simulink model "balancingOptTauQpExtWrenches"  (Simulink 8.3)
settings: Solver=FixedStepDiscrete  StartTime=0.0  StopTime=simulationTime  FixedStep=Ts  RelTol=1e-3
InitFcn:
  | initBalancingOptTauQpExtWrenches;
values from neighbouring files (symbols this model uses):
  activeFeetConstraints = [1 1]    [initBalancingOptTauQpExtWrenches.m]
  noOscillationTime = 0    [initBalancingOptTauQpExtWrenches.m]
  Ts = 0.01    [initBalancingOptTauQpExtWrenches.m]
undefined symbols (not defined in the file or in its folder): bVectorConstraints, ConstraintsMatrix, dampings, directionOfOscillation, DiscIntNeverNeededParam, footSize, gainMomentum, gainsDCOM, gainsICOM, gainsPCOM, impedances, impedencesSat, increasingRatesImp, integralGains, referenceParams, ROBOT_DOF, ROBOT_DOF_FOR_SIMULINK, satIntegral
undefined symbols (not defined in the file): localName, robotName
libraries: WBCLibrary x35, simulink x2
settings Model: Creator=daniele  LastModifiedBy=daniele
settings DataIOCC: SignalLoggingSaveFormat=Dataset
settings OptimizationCC: ExpressionDepthLimit=2147483647
settings DebuggingCC: FcnCallInpInsideContextMsg=EnableAllAsWarning
settings SFSimCC: SimParseCustomCode=off

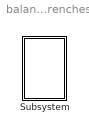
== system balancingOptTauQpExtWrenches ==
  Subsystem : Subsystem  mask{robotName=robotName, Ts=Ts, localName=localName}
      mask prompts: robotName "robot name"; localName "module name"

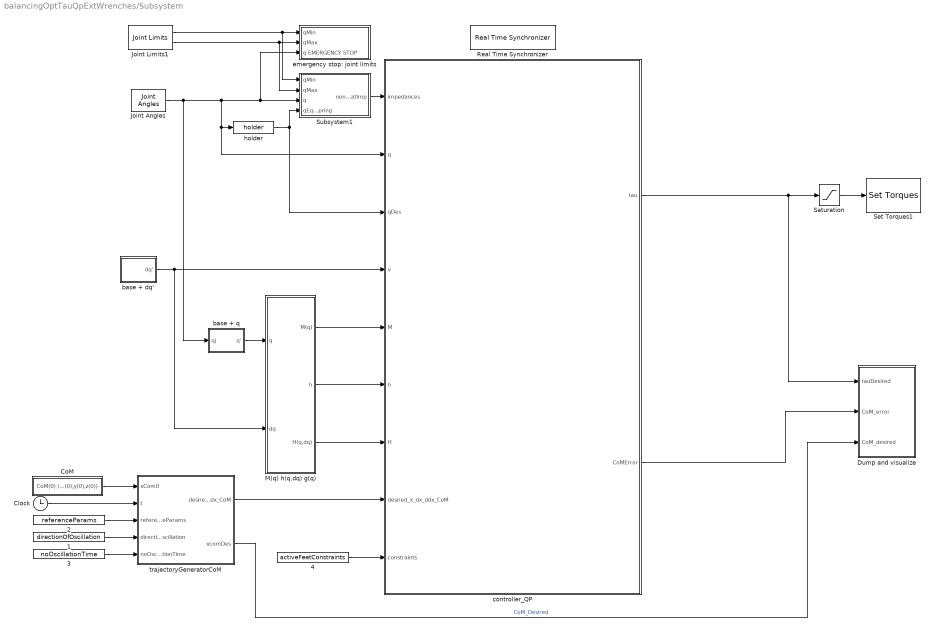
== system balancingOptTauQpExtWrenches/Subsystem ==
  "    1" : Constant  Value=directionOfOscillation
  "    2" : Constant  Value=referenceParams
  "    3" : Constant  Value=noOscillationTime
  "    4" : Constant  Value=activeFeetConstraints
  Clock : Clock
  "CoM " : Subsystem
  Dump and visualize : Subsystem
  Joint Angles : WBCLibrary/wholeBodyStates/Joint Angles  robotName=robotName  localName=localName
  Joint Limits1 : WBCLibrary/wholeBodyModel/Joint Limits  robotName=robotName  localName=localName
  M(q) h(q,dq) g(q) : Subsystem
  Real Time Synchronizer : WBCLibrary/Utilities/Real Time Synchronizer  Priority=-10  threadPeriod=Ts
  Saturation : Saturate  UpperLimit=24  LowerLimit=-24
  Set Torques1 : WBCLibrary/wholeBodyActuators/Set Torques  val=6  robotName=robotName  localName=localName
  Subsystem1 : Subsystem
  base + dq' : Subsystem
  base + q : Subsystem
  controller_QP : Subsystem
  emergency stop: joint limits : Subsystem
  "holder " : WBCLibrary/Utilities/holder 
  trajectoryGeneratorCoM : MATLAB Function  TreatAsAtomicUnit=on
  wires:
  trajectoryGeneratorCoM/1(desired_x_dx_ddx_CoM) -> controller_QP/8(desired_x_dx_ddx_CoM)
  "CoM "/1(CoM(0) (x(0),y(0),z(0))) -> trajectoryGeneratorCoM/1(xCom0)
  base + q/1(q') -> M(q) h(q,dq) g(q)/1(q)
  "holder "/1 -> controller_QP/3(qDes), Subsystem1/4(qEquSpring)
  base + dq'/1(dq') -> M(q) h(q,dq) g(q)/2(dq), controller_QP/4(v)
  M(q) h(q,dq) g(q)/1(M(q)) -> controller_QP/5(M)
  "    2"/1 -> trajectoryGeneratorCoM/3(referenceParams)
  Clock/1 -> trajectoryGeneratorCoM/2(t)
  Subsystem1/1(nonLinSatImp) -> controller_QP/1(impedances)
  Joint Limits1/1 -> emergency stop: joint limits/1(qMin), Subsystem1/1(qMin)
  Joint Limits1/2 -> emergency stop: joint limits/2(qMax), Subsystem1/2(qMax)
  Joint Angles/1 -> base + q/1(qj), controller_QP/2(q), "holder "/1, emergency stop: joint limits/3(q EMERGENCY STOP), Subsystem1/3(q)
  "    1"/1 -> trajectoryGeneratorCoM/4(directionOfOscillation)
  "    3"/1 -> trajectoryGeneratorCoM/5(noOscillationTime)
  M(q) h(q,dq) g(q)/2(h) -> controller_QP/6(h)
  M(q) h(q,dq) g(q)/3(H(q,dq)) -> controller_QP/7(H)
  "    4"/1 -> controller_QP/9(constraints)
  controller_QP/1(tau) -> Dump and visualize/1(tauDesired), Saturation/1
  controller_QP/2(CoMError) -> Dump and visualize/2(CoM_error)
  trajectoryGeneratorCoM/2(xcomDes) -> Dump and visualize/3(CoM_desired)  "CoM_Desired"
  Saturation/1 -> Set Torques1/1

== system balancingOptTauQpExtWrenches/Subsystem/CoM  ==
  "COMFwdKin " : WBCLibrary/wholeBodyModel/Forward Kinematics/COMFwdKin   robotName=robotName  localName=localName
  "CoM6D ->  CoMXYZ" : Selector  InputPortWidth=7  Indices=[1 2 3]
  "holder " : WBCLibrary/Utilities/holder 
  CoM(0) (x(0),y(0),z(0)) : Outport
  wires:
  "COMFwdKin "/1 -> "CoM6D ->  CoMXYZ"/1
  "CoM6D ->  CoMXYZ"/1 -> "holder "/1
  "holder "/1 -> CoM(0) (x(0),y(0),z(0))/1

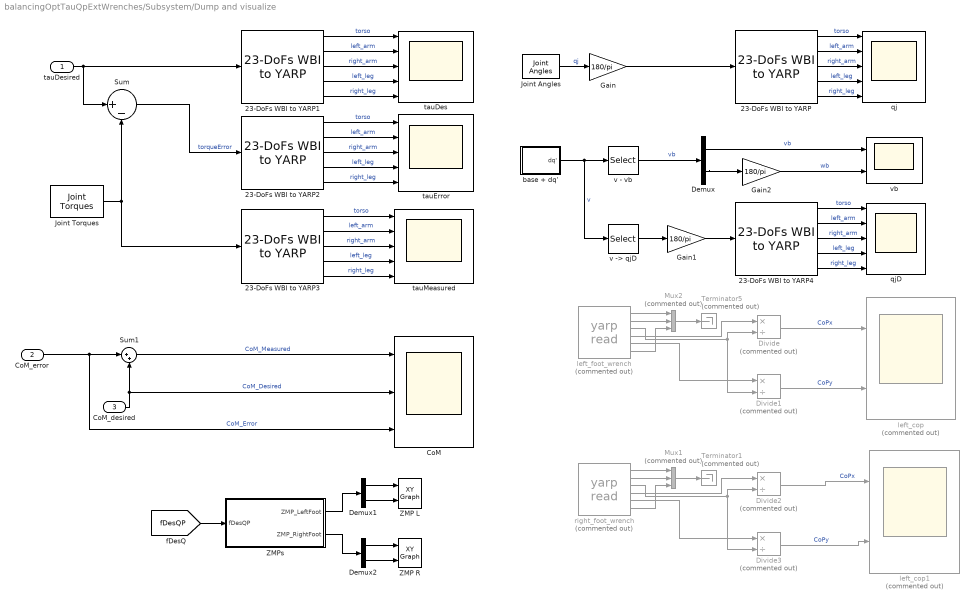
== system balancingOptTauQpExtWrenches/Subsystem/Dump and visualize ==
  tauDesired : Inport
  CoM_error : Inport  Port=2
  CoM_desired : Inport  Port=3
  23-DoFs WBI to YARP{,1..4} (5 alike) : WBCLibrary/Utilities/23-DoFs WBI to YARP
  CoM : Scope  NumInputPorts=3
      settings: ShowLegends=on  TimeRange=400  YMin=-0.2~-0.2~-0.006  YMax=0.5~0.5~0.004  SaveName=CoM_data
  Demux : Demux  Outputs=2
  Demux1 : Demux  Outputs=2
  Demux2 : Demux  Outputs=2
  Divide{,1..3} (4 alike) : Product  Commented=on  Inputs=*/
  Gain : Gain  Gain=180/pi
  Gain1 : Gain  Gain=180/pi
  Gain2 : Gain  Gain=180/pi
  Joint Angles : WBCLibrary/wholeBodyStates/Joint Angles  robotName=robotName  localName=localName
  Joint Torques : WBCLibrary/wholeBodyStates/Joint Torques  robotName=robotName  localName=localName
  Mux1 : Mux  Commented=on  Inputs=3
  Mux2 : Mux  Commented=on  Inputs=3
  Sum : Sum  Inputs=|+-
  Sum1 : Sum  Inputs=|++
  Terminator1 : Terminator  Commented=on
  Terminator5 : Terminator  Commented=on
  ZMP L : simulink/Sinks/XY Graph  xmin=footSize(1,1)  xmax=footSize(1,2)  ymin=footSize(2,1)  ymax=footSize(2,2)  st=-1
  ZMP R : simulink/Sinks/XY Graph  xmin=footSize(1,1)  xmax=footSize(1,2)  ymin=footSize(2,1)  ymax=footSize(2,2)  st=-1
  ZMPs : Subsystem
  base + dq' : Subsystem
  left_cop : Scope  Commented=on  NumInputPorts=2
      settings: ShowLegends=on  TimeRange=42.68  YMin=-50~-20  YMax=250~180  SaveName=ScopeData6
  left_cop1 : Scope  Commented=on  NumInputPorts=2
      settings: ShowLegends=on  TimeRange=42.68  YMin=-50~-20  YMax=250~180  SaveName=ScopeData3
  left_foot_wrench : WBCLibrary/Utilities/yarp read  Commented=on  from=['/wholeBodyDynamicsTree/filtered/l_foot_ft_sensor:o']  to='...'  num=6  blocking=off  timestamp=off  autoconnect=on
  qj : Scope  NumInputPorts=5
      settings: ShowLegends=on  TimeRange=40  YMin=-10~-50~-50~-20~-40  YMax=10~100~100~40~40  SaveName=qj_and_v
  qjD : Scope  NumInputPorts=5
      settings: ShowLegends=on  TimeRange=40  YMin=-15~-10~-20~-20~-20  YMax=20~10~30~20~20  SaveName=qj_and_v1
  right_foot_wrench : WBCLibrary/Utilities/yarp read  Commented=on  from=['/wholeBodyDynamicsTree/filtered/l_foot_ft_sensor:o']  to='...'  num=6  blocking=off  timestamp=off  autoconnect=on
  tauDes : Scope  NumInputPorts=5
      settings: ShowLegends=on  TimeRange=14  YMin=-20~-3~-3~-8~-10  YMax=10~3~3~4~10  SaveName=tauDes
  tauError : Scope  NumInputPorts=5
      settings: ShowLegends=on  TimeRange=90  YMin=-3~-6~-5~-4~-4  YMax=3~6~5~4~6  SaveName=tauError
  tauMeasured : Scope  NumInputPorts=5
      settings: ShowLegends=on  TimeRange=14  YMin=-15~-8~-5~-8~-10  YMax=10~4~5~6~10  SaveName=tauMeasured
  v - vb : Selector  InputPortWidth=ROBOT_DOF+6  Indices=[1:6]
  "v -> qjD" : Selector  InputPortWidth=ROBOT_DOF+6  Indices=[7:ROBOT_DOF+6]
  vb : Scope  NumInputPorts=2
      settings: ShowLegends=on  TimeRange=40  YMin=-0.08~-10  YMax=0.08~10  SaveName=qj_and_v2
  wires:
  CoM_error/1 -> CoM/3, Sum1/1  "CoM_Error"
  tauDesired/1 -> Sum/1, 23-DoFs WBI to YARP1/1
  Joint Torques/1 -> 23-DoFs WBI to YARP3/1, Sum/2
  CoM_desired/1 -> Sum1/2, CoM/2  "CoM_Desired"
  Sum1/1 -> CoM/1  "CoM_Measured"
  base + dq'/1(dq') -> "v -> qjD"/1, v - vb/1  "v"
  Joint Angles/1 -> Gain/1  "qj"
  Gain/1 -> 23-DoFs WBI to YARP/1
  23-DoFs WBI to YARP/5 -> qj/5  "right_leg"
  23-DoFs WBI to YARP/1 -> qj/1  "torso"
  23-DoFs WBI to YARP/2 -> qj/2  "left_arm"
  23-DoFs WBI to YARP/4 -> qj/4  "left_leg"
  23-DoFs WBI to YARP/3 -> qj/3  "right_arm"
  23-DoFs WBI to YARP1/5 -> tauDes/5  "right_leg"
  23-DoFs WBI to YARP1/1 -> tauDes/1  "torso"
  23-DoFs WBI to YARP1/2 -> tauDes/2  "left_arm"
  23-DoFs WBI to YARP1/4 -> tauDes/4  "left_leg"
  23-DoFs WBI to YARP1/3 -> tauDes/3  "right_arm"
  23-DoFs WBI to YARP2/5 -> tauError/5  "right_leg"
  23-DoFs WBI to YARP2/1 -> tauError/1  "torso"
  23-DoFs WBI to YARP2/2 -> tauError/2  "left_arm"
  23-DoFs WBI to YARP2/4 -> tauError/4  "left_leg"
  23-DoFs WBI to YARP2/3 -> tauError/3  "right_arm"
  Sum/1 -> 23-DoFs WBI to YARP2/1  "torqueError"
  23-DoFs WBI to YARP3/5 -> tauMeasured/5  "right_leg"
  23-DoFs WBI to YARP3/1 -> tauMeasured/1  "torso"
  23-DoFs WBI to YARP3/2 -> tauMeasured/2  "left_arm"
  23-DoFs WBI to YARP3/4 -> tauMeasured/4  "left_leg"
  23-DoFs WBI to YARP3/3 -> tauMeasured/3  "right_arm"
  23-DoFs WBI to YARP4/5 -> qjD/5  "right_leg"
  23-DoFs WBI to YARP4/1 -> qjD/1  "torso"
  23-DoFs WBI to YARP4/2 -> qjD/2  "left_arm"
  23-DoFs WBI to YARP4/4 -> qjD/4  "left_leg"
  23-DoFs WBI to YARP4/3 -> qjD/3  "right_arm"
  "v -> qjD"/1 -> Gain1/1
  v - vb/1 -> Demux/1  "vb"
  Demux/1 -> vb/1  "vb"
  Demux/2 -> Gain2/1
  Gain1/1 -> 23-DoFs WBI to YARP4/1
  Gain2/1 -> vb/2  "wb"
  left_foot_wrench/2 -> Mux2/2
  left_foot_wrench/4 -> Divide/1
  left_foot_wrench/5 -> Divide1/1
  left_foot_wrench/6 -> Mux2/3
  left_foot_wrench/3 -> Divide/2, Divide1/2
  left_foot_wrench/1 -> Mux2/1
  Mux2/1 -> Terminator5/1
  Divide/1 -> left_cop/1  "CoPx"
  Divide1/1 -> left_cop/2  "CoPy"
  right_foot_wrench/2 -> Mux1/2
  right_foot_wrench/4 -> Divide2/1
  right_foot_wrench/5 -> Divide3/1
  right_foot_wrench/6 -> Mux1/3
  right_foot_wrench/3 -> Divide2/2, Divide3/2
  right_foot_wrench/1 -> Mux1/1
  Mux1/1 -> Terminator1/1
  Divide2/1 -> left_cop1/1  "CoPx"
  Divide3/1 -> left_cop1/2  "CoPy"
  [fDesQP] -> ZMPs/1(fDesQP)
  ZMPs/1(ZMP_LeftFoot) -> Demux1/1
  ZMPs/2(ZMP_RightFoot) -> Demux2/1
  Demux1/1 -> ZMP L/1
  Demux1/2 -> ZMP L/2
  Demux2/1 -> ZMP R/1
  Demux2/2 -> ZMP R/2

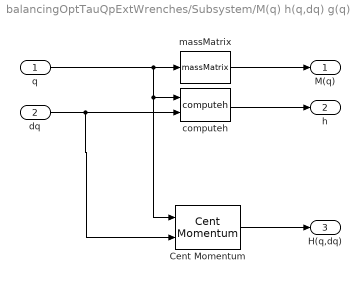
== system balancingOptTauQpExtWrenches/Subsystem/M(q) h(q,dq) g(q) ==
  q : Inport
  dq : Inport  Port=2
  Cent Momentum : WBCLibrary/wholeBodyModel/Dynamics/Cent Momentum  robotName=robotName  localName=localName
  computeh : WBCLibrary/wholeBodyModel/Dynamics/computeh  val=7  robotname=robotName  localname=localName
  massMatrix : WBCLibrary/wholeBodyModel/Dynamics/massMatrix  val=8  robotname=robotName  localname=localName
  M(q) : Outport
  h : Outport  Port=2
  H(q,dq) : Outport  Port=3
  wires:
  computeh/1 -> h/1
  massMatrix/1 -> M(q)/1
  q/1 -> Cent Momentum/1, computeh/1, massMatrix/1
  dq/1 -> Cent Momentum/2, computeh/2
  Cent Momentum/1 -> H(q,dq)/1

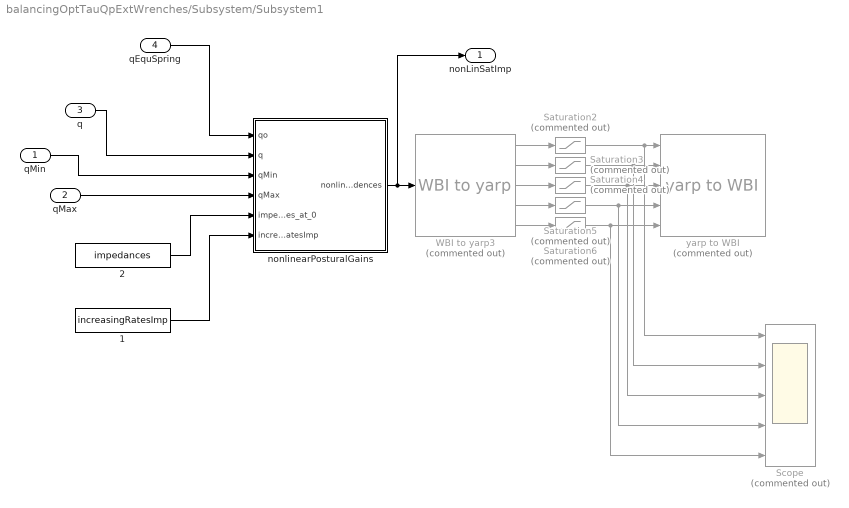
== system balancingOptTauQpExtWrenches/Subsystem/Subsystem1 ==
  qMin : Inport
  qMax : Inport  Port=2
  q : Inport  Port=3
  qEquSpring : Inport  Port=4
  "    1" : Constant  Value=increasingRatesImp
  "    2" : Constant  Value=impedances
  Saturation2 : Saturate  Commented=on  UpperLimit=impedencesSat(1)  LowerLimit=0  SampleTime=Ts
  Saturation3 : Saturate  Commented=on  UpperLimit=impedencesSat(2)  LowerLimit=0  SampleTime=Ts
  Saturation4 : Saturate  Commented=on  UpperLimit=impedencesSat(2)  LowerLimit=0  SampleTime=Ts
  Saturation5 : Saturate  Commented=on  UpperLimit=impedencesSat(3)  LowerLimit=0  SampleTime=Ts
  Saturation6 : Saturate  Commented=on  UpperLimit=impedencesSat(3)  LowerLimit=0  SampleTime=Ts
  Scope : Scope  Commented=on  NumInputPorts=5
      settings: ShowLegends=on  TimeRange=12  YMin=-5~-5~-5~0.9370629370629331~-5  YMax=5~5~5~4.937062937062933~5
  WBI to yarp3 : WBCLibrary/Utilities/WBI to yarp  Commented=on
  "nonlinearPosturalGains " : MATLAB Function  TreatAsAtomicUnit=on
  yarp to WBI : WBCLibrary/Utilities/yarp to WBI  Commented=on
  nonLinSatImp : Outport
  wires:
  WBI to yarp3/1 -> Saturation2/1
  WBI to yarp3/2 -> Saturation3/1
  WBI to yarp3/3 -> Saturation4/1
  WBI to yarp3/4 -> Saturation5/1
  WBI to yarp3/5 -> Saturation6/1
  "nonlinearPosturalGains "/1(nonlinearImpedences) -> nonLinSatImp/1, WBI to yarp3/1
  qEquSpring/1 -> "nonlinearPosturalGains "/1(qo)
  qMin/1 -> "nonlinearPosturalGains "/3(qMin)
  qMax/1 -> "nonlinearPosturalGains "/4(qMax)
  "    2"/1 -> "nonlinearPosturalGains "/5(impedences_at_0)
  "    1"/1 -> "nonlinearPosturalGains "/6(increasingRatesImp)
  q/1 -> "nonlinearPosturalGains "/2(q)
  Saturation6/1 -> Scope/5, yarp to WBI/5
  Saturation4/1 -> Scope/3, yarp to WBI/3
  Saturation5/1 -> Scope/4, yarp to WBI/4
  Saturation3/1 -> Scope/2, yarp to WBI/2
  Saturation2/1 -> Scope/1, yarp to WBI/1

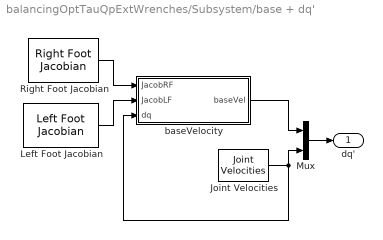
== system balancingOptTauQpExtWrenches/Subsystem/base + dq' ==
  Joint Velocities : WBCLibrary/wholeBodyStates/Joint Velocities  robotName=robotName  localName=localName
  Left Foot Jacobian : WBCLibrary/wholeBodyModel/Jacobians/Left Foot Jacobian  robotName=robotName  localName=localName
  Mux : Mux  Inputs=2
  Right Foot Jacobian : WBCLibrary/wholeBodyModel/Jacobians/Right Foot Jacobian  robotName=robotName  localName=localName
  baseVelocity : Subsystem  AncestorBlock=WBCLibrary/Utilities/baseVelocity  mask(baseVelocity){}
      mask help: This block computes the velocity of the floating base of a bipedal robot
  dq' : Outport
  wires:
  Left Foot Jacobian/1 -> baseVelocity/2(JacobLF)
  Right Foot Jacobian/1 -> baseVelocity/1(JacobRF)
  baseVelocity/1(baseVel) -> Mux/1
  Joint Velocities/1 -> baseVelocity/3(dq), Mux/2
  Mux/1 -> dq'/1

== system balancingOptTauQpExtWrenches/Subsystem/base + q ==
  qj : Inport
  Constant1 : Constant  Value=zeros(16,1)
  Mux : Mux  Inputs=2
  q' : Outport
  wires:
  Mux/1 -> q'/1
  qj/1 -> Mux/2
  Constant1/1 -> Mux/1

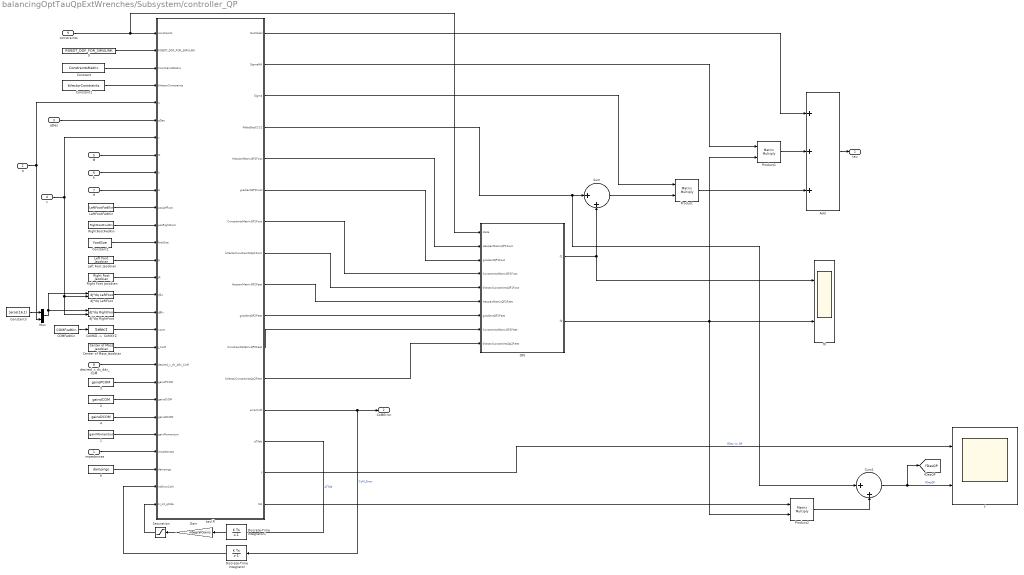
== system balancingOptTauQpExtWrenches/Subsystem/controller_QP ==
  impedances : Inport
  q : Inport  Port=2
  qDes : Inport  Port=3
  v : Inport  Port=4
  M : Inport  Port=5
  h : Inport  Port=6
  H : Inport  Port=7
  desired_x_dx_ddx_CoM : Inport  Port=8
  constraints : Inport  Port=9
  "    1" : Constant  Value=gainMomentum
  "    2" : Constant  Value=gainsICOM
  "    3" : Constant  Value=gainsPCOM
  "    4" : Constant  Value=gainsDCOM
  "    5" : Constant  Value=ROBOT_DOF_FOR_SIMULINK
  "    6" : Constant  Value=dampings
  Add : Sum  Inputs=+++
  "COMFwdKin " : WBCLibrary/wholeBodyModel/Forward Kinematics/COMFwdKin   robotName=robotName  localName=localName
  Center of Mass Jacobian : WBCLibrary/wholeBodyModel/Jacobians/Center of Mass Jacobian  robotName=robotName  localName=localName
  "CoM6D ->  CoMXYZ" : Selector  InputPortWidth=7  Indices=[1 2 3]
  Constant : Constant  Value=ConstraintsMatrix
  Constant1 : Constant  Value=bVectorConstraints
  Constant2 : Constant  Value=footSize
  Constant3 : Constant  Value=zeros(16,1)
  Discrete-Time Integrator : DiscreteIntegrator  InitialCondition=[0 0 0]  SampleTime=Ts  ICPrevOutput=DiscIntNeverNeededParam  ICPrevScaledInput=DiscIntNeverNeededParam
  Discrete-Time Integrator1 : DiscreteIntegrator  InitialCondition=zeros(ROBOT_DOF,1)  SampleTime=Ts  ICPrevOutput=DiscIntNeverNeededParam  ICPrevScaledInput=DiscIntNeverNeededParam
  Gain : Gain  Gain=integralGains
  Left Foot Jacobian : WBCLibrary/wholeBodyModel/Jacobians/Left Foot Jacobian  robotName=robotName  localName=localName
  LeftFootFwdKin : WBCLibrary/wholeBodyModel/Forward Kinematics/LeftFootFwdKin  robotName=robotName  localName=localName
  Mux : Mux  Inputs=2
  Product : Product  Multiplication=Matrix(*)
  Product1 : Product  Multiplication=Matrix(*)
  Product2 : Product  Multiplication=Matrix(*)
  QPs : Subsystem
  Right Foot Jacobian : WBCLibrary/wholeBodyModel/Jacobians/Right Foot Jacobian  robotName=robotName  localName=localName
  RightFootFwdKin : WBCLibrary/wholeBodyModel/Forward Kinematics/RightFootFwdKin  robotName=robotName  localName=localName
  Saturation : Saturate  UpperLimit=satIntegral  LowerLimit=-satIntegral
  Sum : Sum  Inputs=|++
  Sum1 : Sum  Inputs=|++
  dJ*dq LeftFoot : WBCLibrary/wholeBodyModel/Dynamics/dJ*dq LeftFoot  val=9  robotName=robotName  localName=localName
  dJ*dq RightFoot : WBCLibrary/wholeBodyModel/Dynamics/dJ*dq RightFoot  val=9  robotName=robotName  localName=localName
  f : Scope  NumInputPorts=2
      settings: TimeRange=40  YMin=-50~-50  YMax=200~200  SaveName=ScopeData2
  f0 : Scope  NumInputPorts=2
      settings: TimeRange=25  YMin=-30~-30  YMax=30~30
  "tau(f) " : MATLAB Function  TreatAsAtomicUnit=on
  tau : Outport
  CoMError : Outport  Port=2
  tag scope: fDesQP=global
  wires:
  constraints/1 -> QPs/1(state), "tau(f) "/1(constraints)
  Discrete-Time Integrator/1 -> "tau(f) "/27(intErrorCoM)
  "tau(f) "/13(errorCoM) -> CoMError/1, Discrete-Time Integrator/1  "CoM_Error"
  Discrete-Time Integrator1/1 -> Gain/1
  "tau(f) "/14(qTilde) -> Discrete-Time Integrator1/1  "qTilde"
  Gain/1 -> Saturation/1
  Saturation/1 -> "tau(f) "/28(ki_int_qtilde)
  q/1 -> Mux/2, "tau(f) "/5(q)
  qDes/1 -> "tau(f) "/6(qDes)
  M/1 -> "tau(f) "/8(M)
  h/1 -> "tau(f) "/9(h)
  desired_x_dx_ddx_CoM/1 -> "tau(f) "/20(desired_x_dx_ddx_CoM)
  impedances/1 -> "tau(f) "/25(impedances)
  H/1 -> "tau(f) "/10(H)
  "    6"/1 -> "tau(f) "/26(dampings)
  v/1 -> dJ*dq RightFoot/2, dJ*dq LeftFoot/2, "tau(f) "/7(v)
  Mux/1 -> dJ*dq LeftFoot/1, dJ*dq RightFoot/1
  "COMFwdKin "/1 -> "CoM6D ->  CoMXYZ"/1
  RightFootFwdKin/1 -> "tau(f) "/12(posRightFoot)
  LeftFootFwdKin/1 -> "tau(f) "/11(posLefFoot)
  Left Foot Jacobian/1 -> "tau(f) "/14(JL)
  Right Foot Jacobian/1 -> "tau(f) "/15(JR)
  dJ*dq LeftFoot/1 -> "tau(f) "/16(dJLv)
  Constant3/1 -> Mux/1
  dJ*dq RightFoot/1 -> "tau(f) "/17(dJRv)
  "CoM6D ->  CoMXYZ"/1 -> "tau(f) "/18(xcom)
  Center of Mass Jacobian/1 -> "tau(f) "/19(J_CoM)
  "    3"/1 -> "tau(f) "/21(gainsPCOM)
  "    2"/1 -> "tau(f) "/22(gainsICOM)
  "    4"/1 -> "tau(f) "/23(gainsDCOM)
  "    1"/1 -> "tau(f) "/24(gainMomentum)
  "tau(f) "/5(HessianMatrixQP1Foot) -> QPs/2(HessianMatrixQP1Foot)
  "tau(f) "/6(gradientQP1Foot) -> QPs/3(gradientQP1Foot)
  "tau(f) "/9(HessianMatrixQP2Feet) -> QPs/6(HessianMatrixQP2Feet)
  "tau(f) "/10(gradientQP2Feet) -> QPs/7(gradientQP2Feet)
  "tau(f) "/11(ConstraintsMatrixQP2Feet) -> QPs/8(ConstraintsMatrixQP2Feet)
  "tau(f) "/12(bVectorConstraintsQp2Feet) -> QPs/9(bVectorConstraintsQp2Feet)
  "tau(f) "/4(fHdotDesC1C2) -> Sum1/1, Sum/1
  QPs/1(f1) -> Sum/2, f0/1
  "tau(f) "/3(Sigma) -> Product/1
  Sum/1 -> Product/2
  "tau(f) "/2(SigmaNA) -> Product1/1
  QPs/2(f0) -> Product1/2, Product2/2, f0/2
  Product1/1 -> Add/2
  Product/1 -> Add/3
  "tau(f) "/1(tauModel) -> Add/1
  Add/1 -> tau/1
  "tau(f) "/16(NA) -> Product2/1
  Product2/1 -> Sum1/2
  "tau(f) "/15(f) -> f/1  "fDes no QP"
  Sum1/1 -> [fDesQP], f/2  "fDesQP"
  "    5"/1 -> "tau(f) "/2(ROBOT_DOF_FOR_SIMULINK)
  Constant/1 -> "tau(f) "/3(ConstraintsMatrix)
  Constant1/1 -> "tau(f) "/4(bVectorConstraints)
  "tau(f) "/7(ConstraintsMatrixQP1Foot) -> QPs/4(ConstraintsMatrixQP1Foot)
  "tau(f) "/8(bVectorConstraintsQp1Foot) -> QPs/5(bVectorConstraintsQP1Foot)
  Constant2/1 -> "tau(f) "/13(footSize)

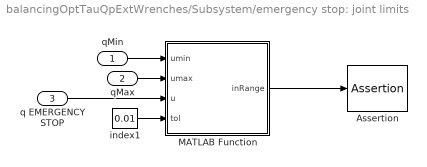
== system balancingOptTauQpExtWrenches/Subsystem/emergency stop: joint limits ==
  qMin : Inport
  qMax : Inport  Port=2
  q EMERGENCY STOP : Inport  Port=3
  Assertion : Assertion
  MATLAB Function : MATLAB Function  TreatAsAtomicUnit=on
  index1 : Constant  Value=0.01  VectorParams1D=off
  wires:
  qMin/1 -> MATLAB Function/1(umin)
  qMax/1 -> MATLAB Function/2(umax)
  index1/1 -> MATLAB Function/4(tol)
  q EMERGENCY STOP/1 -> MATLAB Function/3(u)
  MATLAB Function/1(inRange) -> Assertion/1

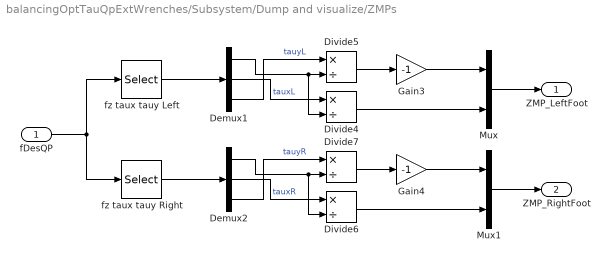
== system balancingOptTauQpExtWrenches/Subsystem/Dump and visualize/ZMPs ==
  fDesQP : Inport
  Demux1 : Demux  Outputs=3
  Demux2 : Demux  Outputs=3
  Divide{4..7} (4 alike) : Product  Inputs=*/
  Gain3 : Gain  Gain=-1
  Gain4 : Gain  Gain=-1
  Mux : Mux  Inputs=2
  Mux1 : Mux  Inputs=2
  fz taux tauy Left : Selector  InputPortWidth=12  Indices=[3 4 5]
  fz taux tauy Right : Selector  InputPortWidth=12  Indices=[9 10 11]
  ZMP_LeftFoot : Outport
  ZMP_RightFoot : Outport  Port=2
  wires:
  fz taux tauy Left/1 -> Demux1/1
  Demux1/1 -> Divide4/2, Divide5/2
  Divide7/1 -> Gain4/1
  Divide4/1 -> Mux/2
  Divide5/1 -> Gain3/1
  fz taux tauy Right/1 -> Demux2/1
  Demux2/1 -> Divide6/2, Divide7/2
  fDesQP/1 -> fz taux tauy Left/1, fz taux tauy Right/1
  Gain3/1 -> Mux/1
  Mux/1 -> ZMP_LeftFoot/1
  Divide6/1 -> Mux1/2
  Gain4/1 -> Mux1/1
  Mux1/1 -> ZMP_RightFoot/1
  Demux1/2 -> Divide4/1  "tauxL"
  Demux1/3 -> Divide5/1  "tauyL"
  Demux2/2 -> Divide6/1  "tauxR"
  Demux2/3 -> Divide7/1  "tauyR"

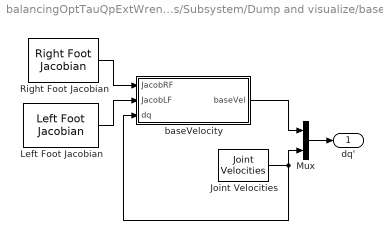
== system balancingOptTauQpExtWrenches/Subsystem/Dump and visualize/base + dq' ==
  Joint Velocities : WBCLibrary/wholeBodyStates/Joint Velocities  robotName=robotName  localName=localName
  Left Foot Jacobian : WBCLibrary/wholeBodyModel/Jacobians/Left Foot Jacobian  robotName=robotName  localName=localName
  Mux : Mux  Inputs=2
  Right Foot Jacobian : WBCLibrary/wholeBodyModel/Jacobians/Right Foot Jacobian  robotName=robotName  localName=localName
  baseVelocity : Subsystem  AncestorBlock=WBCLibrary/Utilities/baseVelocity  mask(baseVelocity){}
      mask help: This block computes the velocity of the floating base of a bipedal robot
  dq' : Outport
  wires:
  Left Foot Jacobian/1 -> baseVelocity/2(JacobLF)
  Right Foot Jacobian/1 -> baseVelocity/1(JacobRF)
  baseVelocity/1(baseVel) -> Mux/1
  Joint Velocities/1 -> baseVelocity/3(dq), Mux/2
  Mux/1 -> dq'/1

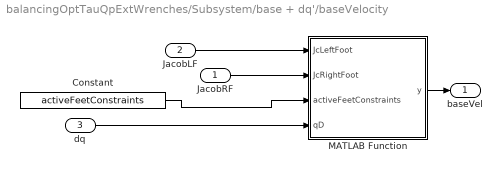
== system balancingOptTauQpExtWrenches/Subsystem/base + dq'/baseVelocity ==
  JacobRF : Inport
  JacobLF : Inport  Port=2
  dq : Inport  Port=3
  Constant : Constant  Value=activeFeetConstraints
  MATLAB Function : MATLAB Function  TreatAsAtomicUnit=on
  baseVel : Outport
  wires:
  JacobLF/1 -> MATLAB Function/1(JcLeftFoot)
  JacobRF/1 -> MATLAB Function/2(JcRightFoot)
  MATLAB Function/1(y) -> baseVel/1
  dq/1 -> MATLAB Function/4(qD)
  Constant/1 -> MATLAB Function/3(activeFeetConstraints)

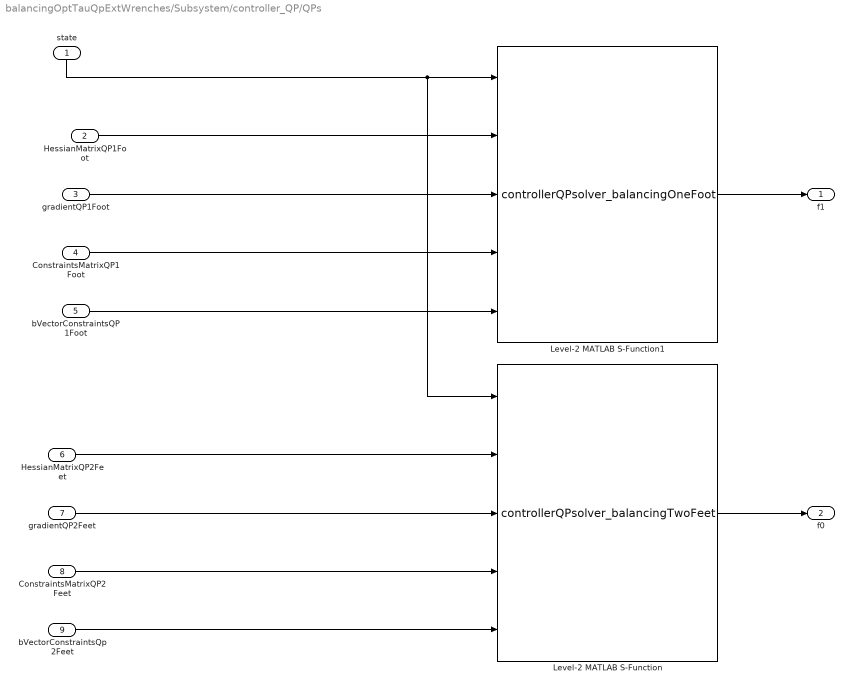
== system balancingOptTauQpExtWrenches/Subsystem/controller_QP/QPs ==
  state : Inport
  HessianMatrixQP1Foot : Inport  Port=2
  gradientQP1Foot : Inport  Port=3
  ConstraintsMatrixQP1Foot : Inport  Port=4
  bVectorConstraintsQP1Foot : Inport  Port=5
  HessianMatrixQP2Feet : Inport  Port=6
  gradientQP2Feet : Inport  Port=7
  ConstraintsMatrixQP2Feet : Inport  Port=8
  bVectorConstraintsQp2Feet : Inport  Port=9
  Level-2 MATLAB S-Function : M-S-Function  FunctionName=controllerQPsolver_balancingTwoFeet
  Level-2 MATLAB S-Function1 : M-S-Function  FunctionName=controllerQPsolver_balancingOneFoot
  f1 : Outport
  f0 : Outport  Port=2
  wires:
  state/1 -> Level-2 MATLAB S-Function/1, Level-2 MATLAB S-Function1/1
  gradientQP2Feet/1 -> Level-2 MATLAB S-Function/3
  HessianMatrixQP1Foot/1 -> Level-2 MATLAB S-Function1/2
  ConstraintsMatrixQP2Feet/1 -> Level-2 MATLAB S-Function/4
  gradientQP1Foot/1 -> Level-2 MATLAB S-Function1/3
  HessianMatrixQP2Feet/1 -> Level-2 MATLAB S-Function/2
  Level-2 MATLAB S-Function/1 -> f0/1
  bVectorConstraintsQp2Feet/1 -> Level-2 MATLAB S-Function/5
  Level-2 MATLAB S-Function1/1 -> f1/1
  ConstraintsMatrixQP1Foot/1 -> Level-2 MATLAB S-Function1/4
  bVectorConstraintsQP1Foot/1 -> Level-2 MATLAB S-Function1/5

== system balancingOptTauQpExtWrenches/Subsystem/Dump and visualize/base + dq'/baseVelocity ==
  JacobRF : Inport
  JacobLF : Inport  Port=2
  dq : Inport  Port=3
  Constant : Constant  Value=activeFeetConstraints
  MATLAB Function : MATLAB Function  TreatAsAtomicUnit=on
  baseVel : Outport
  wires:
  JacobLF/1 -> MATLAB Function/1(JcLeftFoot)
  JacobRF/1 -> MATLAB Function/2(JcRightFoot)
  MATLAB Function/1(y) -> baseVel/1
  dq/1 -> MATLAB Function/4(qD)
  Constant/1 -> MATLAB Function/3(activeFeetConstraints)

== matlab function Subsystem/trajectoryGeneratorCoM ==
  data: desired_x_dx_ddx_CoM output double; xCom0 input double; t input double; referenceParams input double; directionOfOscillation input double; noOscillationTime input double; xcomDes output double
function [desired_x_dx_ddx_CoM,xcomDes]  = fcn(xCom0,t,referenceParams,directionOfOscillation,noOscillationTime)
%#codegen


if t > noOscillationTime
    A = referenceParams(1);
else
    A = 0;
end
f = referenceParams(2);

xcomDes    = xCom0 + A*sin(2*pi*f*t)*directionOfOscillation;
% xcomDes(1) =  xcomDes(1) + 0.01;
xDcomDes   =         A*2*pi*f*cos(2*pi*f*t)*directionOfOscillation;
xDDcomDes  =        -A*(2*pi*f)^2*sin(2*pi*f*t)*directionOfOscillation;

desired_x_dx_ddx_CoM = [xcomDes,xDcomDes,xDDcomDes];

== matlab function Subsystem/base + dq'/baseVelocity/MATLAB Function ==
  data: JcLeftFoot input double; JcRightFoot input double; activeFeetConstraints input double; y output double; qD input double
function y = fcn(JcLeftFoot,JcRightFoot,activeFeetConstraints,qD)
%#codegen
if sum(activeFeetConstraints) == 2
    Jc = [JcLeftFoot;JcRightFoot];
else
    Jc = JcLeftFoot;
end
y = -pinv(Jc(:,1:6))*Jc(:,7:end)*qD;

== matlab function Subsystem/Dump and visualize/base + dq'/baseVelocity/MATLAB Function ==
  data: JcLeftFoot input double; JcRightFoot input double; activeFeetConstraints input double; y output double; qD input double
function y = fcn(JcLeftFoot,JcRightFoot,activeFeetConstraints,qD)
%#codegen
if sum(activeFeetConstraints) == 2
    Jc = [JcLeftFoot;JcRightFoot];
else
    Jc = JcLeftFoot;
end
y = -pinv(Jc(:,1:6))*Jc(:,7:end)*qD;

== matlab function Subsystem/emergency stop: joint limits/MATLAB Function ==
  data: umin input double; umax input double; u input double; inRange output double; tol input double
function inRange = checkRange(umin, umax, u, tol)
%#codegen

res = u < umin + tol | u > umax - tol;
res = sum(res);
if res==0
    inRange = 1;
else
    inRange = 0;
    u < umin + tol | u > umax - tol
end

== matlab function Subsystem/controller_QP/tau(f)  ==
  data: tauModel output double; SigmaNA output double; Sigma output double; fHdotDesC1C2 output double; HessianMatrixQP1Foot output double; gradientQP1Foot output double; ConstraintsMatrixQP1Foot output double; bVectorConstraintsQp1Foot output double; HessianMatrixQP2Feet output double; gradientQP2Feet output double; ConstraintsMatrixQP2Feet output double; bVectorConstraintsQp2Feet output double; constraints input double; ROBOT_DOF_FOR_SIMULINK input double; ConstraintsMatrix input double; bVectorConstraints input double; q input double; qDes input double; v input double; M input double; h input double; H input double; posLefFoot input double; posRightFoot input double; footSize input double; JL input double; JR input double; dJLv input double; dJRv input double; xcom input double; J_CoM input double; desired_x_dx_ddx_CoM input double; gainsPCOM input double; gainsICOM input double; gainsDCOM input double; gainMomentum input double; impedances input double; dampings input double; intErrorCoM input double; ki_int_qtilde input double; errorCoM output double; qTilde output double; f output double; NA output double
function [tauModel,SigmaNA,Sigma,fHdotDesC1C2, ...
          HessianMatrixQP1Foot,gradientQP1Foot,ConstraintsMatrixQP1Foot,bVectorConstraintsQp1Foot,...
          HessianMatrixQP2Feet,gradientQP2Feet,ConstraintsMatrixQP2Feet,bVectorConstraintsQp2Feet,...
          errorCoM,qTilde,f,NA]    =  ...
          controllerFCN(constraints,ROBOT_DOF_FOR_SIMULINK,ConstraintsMatrix,bVectorConstraints,...
          q,qDes,v, M, h, H, posLefFoot, posRightFoot,footSize, JL,JR, dJLv,dJRv, xcom,J_CoM, desired_x_dx_ddx_CoM,...
          gainsPCOM,gainsICOM,gainsDCOM,gainMomentum, impedances,dampings, intErrorCoM,ki_int_qtilde)
%#codegen
e1              = [1;0;0];
e2              = [0;1;0];
e3              = [0;0;1]; 
ROBOT_DOF       = size(ROBOT_DOF_FOR_SIMULINK,1);
PINV_TOL        = 1e-5;
reg             = 0.01;
regHessiansQP   = 1e-7;
gravAcc         = 9.81;
m               = M(1,1);
Mb              = M(1:6,1:6);
Mbj             = M(1:6,7:end);
% Mj              = M(7:end,7:end);

St              = [  zeros(6,ROBOT_DOF);
                   eye(ROBOT_DOF,ROBOT_DOF)];
grav            = [ zeros(2,1);
                   -m*gravAcc;
                    zeros(3,1)];
                
pos_leftFoot   = posLefFoot(1:3);
rotMatLeftFoot = Rf(posLefFoot(4:7));

pos_rightFoot   = posRightFoot(1:3);
rotMatRightFoot = Rf(posRightFoot(4:7));


xDcom           = J_CoM(1:3,:)*v;
qD              = v(7:end);
xDDcomStar      = desired_x_dx_ddx_CoM(:,3) - gainsPCOM*(xcom - desired_x_dx_ddx_CoM(:,1)) - gainsICOM*intErrorCoM - gainsDCOM*(xDcom - desired_x_dx_ddx_CoM(:,2));
Pr              = pos_rightFoot - xcom; % Application point of the contact force on the right foot w.r.t. CoM
Pl              = pos_leftFoot  - xcom; % Application point of the contact force on the left foot w.r.t. CoM


AL = [ eye(3),   zeros(3);
       Sf(Pl),  eye(3)];
AR = [ eye(3), zeros(3);
        Sf(Pr), eye(3) ];
    
A    = [ AL, AR];

Jc   = [ JL*constraints(1) ;
         JR*constraints(2)];
JcDv = [ dJLv*constraints(1) ;
         dJRv*constraints(2)];

JcMinv          = Jc/M;
JcMinvSt        = JcMinv*St;
JcMinvJct       = JcMinv*transpose(Jc);

pinvA         = pinv( A, PINV_TOL)*constraints(1)*constraints(2) + [inv(AL);zeros(6)]*constraints(1)*(1-constraints(2)) + [zeros(6);inv(AR)]*constraints(2)*(1-constraints(1)); 
% PInv_JcMinvSt = pinv( JcMinvSt, PINV_TOL);
PInv_JcMinvSt = JcMinvSt'/(JcMinvSt*JcMinvSt' + reg*eye(size(JcMinvSt,1)));
  
HDotDes  = [ m*xDDcomStar ;
            -gainMomentum*H(4:end)]; 
         

NL        = eye(ROBOT_DOF) - PInv_JcMinvSt*JcMinvSt;

f_HDot           = pinvA*(HDotDes - grav);

fHdotDesC1C2     =  f_HDot*constraints(1)*constraints(2);

NA               =  eye(12,12)-pinvA*A;
JBar             = transpose(Jc(:,7:end)) - Mbj'/Mb*transpose(Jc(:,1:6)); % multiplier of f in tau0

qTilde           =  q-qDes;


Sigma            = -(PInv_JcMinvSt*JcMinvJct + NL*JBar);
SigmaNA          = Sigma*NA;

tauModel         = PInv_JcMinvSt*(JcMinv*h - JcDv) + NL*(h(7:end) - Mbj'/Mb*h(1:6) - diag(impedances)*qTilde  -ki_int_qtilde -diag(dampings)*NL*qD);

CL               = ConstraintsMatrix; 
CL(end-4,1:3)    = -e3'*rotMatLeftFoot;                
CL(end-3,:)      = [ footSize(1,1)*e3'*rotMatLeftFoot', e2'*rotMatLeftFoot'];
CL(end-2,:)      = [-footSize(1,2)*e3'*rotMatLeftFoot',-e2'*rotMatLeftFoot'];

CL(end-1,:)      = [ footSize(2,1)*e3'*rotMatLeftFoot',-e1'*rotMatLeftFoot'];
CL(end  ,:)      = [-footSize(2,2)*e3'*rotMatLeftFoot', e1'*rotMatLeftFoot'];

CR               = ConstraintsMatrix;
CR(end-4,1:3)    = -e3'*rotMatRightFoot;  
CR(end-3,:)      = [ footSize(1,1)*e3'*rotMatRightFoot', e2'*rotMatRightFoot'];
CR(end-2,:)      = [-footSize(1,2)*e3'*rotMatRightFoot',-e2'*rotMatRightFoot'];

CR(end-1,:)      = [ footSize(2,1)*e3'*rotMatRightFoot',-e1'*rotMatRightFoot'];
CR(end  ,:)      = [-footSize(2,2)*e3'*rotMatRightFoot', e1'*rotMatRightFoot'];


ConstraintsMatrix2Feet   = blkdiag(CL,CR);
bVectorConstraints2Feet  = [bVectorConstraints;bVectorConstraints];

ConstraintsMatrixQP1Foot = constraints(1) * (1 - constraints(2)) * CL + ...
                           constraints(2) * (1 - constraints(1)) * CR;
bVectorConstraintsQp1Foot= bVectorConstraints;

ConstraintsMatrixQP2Feet  = ConstraintsMatrix2Feet*NA;
bVectorConstraintsQp2Feet = bVectorConstraints2Feet-ConstraintsMatrix2Feet*f_HDot;

HessianMatrixQP2Feet      = SigmaNA'*SigmaNA + eye(size(SigmaNA,2))*regHessiansQP;
gradientQP2Feet           = SigmaNA'*(tauModel + Sigma*f_HDot);

A1Foot                    = AL*constraints(1)*(1-constraints(2)) + AR*constraints(2)*(1-constraints(1));
HessianMatrixQP1Foot      = A1Foot'*A1Foot + eye(size(A1Foot,2))*regHessiansQP;
gradientQP1Foot           = -A1Foot'*(HDotDes + grav);

f0                        = -pinv(SigmaNA)*(tauModel + Sigma*f_HDot);

f                         = f_HDot + NA*f0;

errorCoM = xcom - desired_x_dx_ddx_CoM(:,1);

== matlab function Subsystem/Subsystem1/nonlinearPosturalGains  ==
  data: qo input double; nonlinearImpedences output double; q input double; qMin input double; qMax input double; impedences_at_0 input double; increasingRatesImp input double
function nonlinearImpedences = fcn(qo,q,qMin,qMax,impedences_at_0,increasingRatesImp)
    %#codegen

    tp =  pi./(2*(qMax-qo));
    tn = -pi./(2*(qMin-qo));

    qTilde = q - qo;
            
    nonlinearImpedences = impedences_at_0' + (increasingRatesImp.*tan((tp.*stepFcn(qTilde) + tn.*stepFcn(-qTilde)).*qTilde).^2)' ;
end

function y = stepFcn(x) 
   %#codegen
   y = x > 0; 
end
